simulink model "bug1"  (R2021b)
settings: Solver=VariableStepAuto  StartTime=0.0  StopTime=10.0  RelTol=1e-3
settings Model: SimulationMode=accelerator  Creator=cemery  LastModifiedBy=cemery

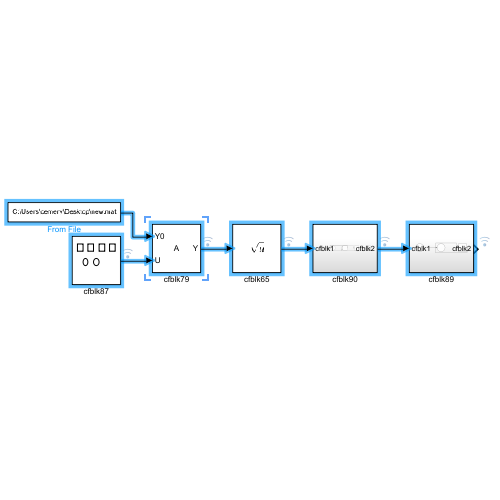
[thumbnail: Simulink's stored preview of the top-level diagram]
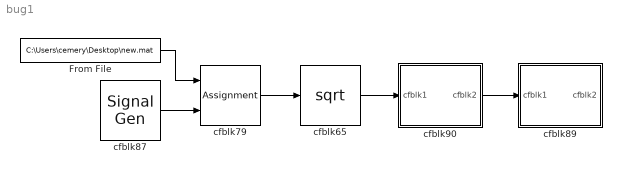
== system bug1 ==
  From File : FromFile  FileName=C:\Users\cemery\Desktop\new.mat  SampleTime=0
  cfblk65 : Sqrt  SaturateOnIntegerOverflow=on
  cfblk79 : Assignment  DiagnosticForDimensions=Warning  IndexOptions=Index vector (dialog)  Indices=1  OutputSizes=1
  cfblk87 : SignalGenerator  WaveForm=square  Amplitude=[478990331.282242]  Units=rad/sec
  cfblk89 : Subsystem
  cfblk90 : Subsystem
  wires:
  From File/1 -> cfblk79/1
  cfblk87/1 -> cfblk79/2
  cfblk79/1 -> cfblk65/1
  cfblk90/1(cfblk2) -> cfblk89/1(cfblk1)
  cfblk65/1 -> cfblk90/1(cfblk1)

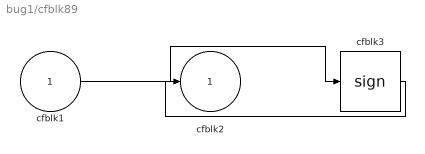
== system bug1/cfblk89 ==
  cfblk1 : Inport
  cfblk3 : Signum
  cfblk2 : Outport
  wires:
  cfblk1/1 -> cfblk3/1
  cfblk3/1 -> cfblk2/1

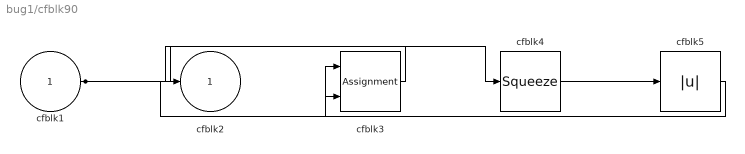
== system bug1/cfblk90 ==
  cfblk1 : Inport
  cfblk3 : Assignment  DiagnosticForDimensions=Warning  IndexOptions=Index vector (dialog)  Indices=1  OutputSizes=1
  cfblk4 : Squeeze
  cfblk5 : Abs
  cfblk2 : Outport
  wires:
  cfblk1/1 -> cfblk4/1, cfblk3/2
  cfblk4/1 -> cfblk5/1
  cfblk5/1 -> cfblk3/1
  cfblk3/1 -> cfblk2/1
